simulink model "FuelCell5"  (R2016b)
settings: Solver=ode45  StartTime=0.0  StopTime=100.0  RelTol=1e-3
undefined symbols (not defined in the file): A, B, C, J, Jmax, lam, n, Rc, Tr
libraries: simulink x1
settings Model: Creator=Kelly  LastModifiedBy=Kelly

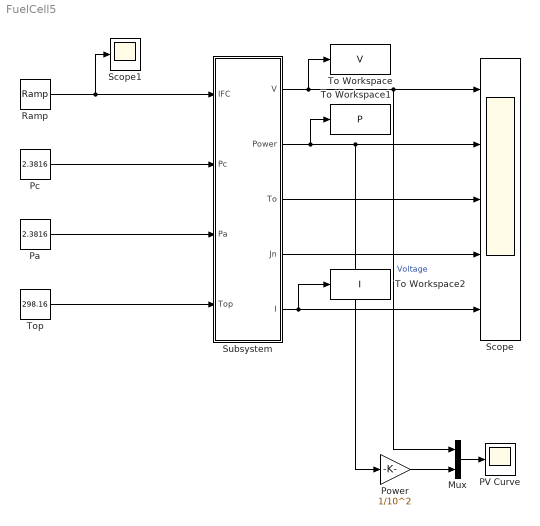
== system FuelCell5 ==
  Mux : Mux  Inputs=2
  PV Curve : Scope
  Pa : Constant  Value=2.3816
  Pc : Constant  Value=2.3816
  Power : Gain  Gain=1/10^2
  Ramp : simulink/Sources/Ramp  slope=Jmax*A/100  start=0  X0=J*A/100
  Scope : Scope  NumInputPorts=5
  Scope1 : Scope
  Subsystem : Subsystem
  To Workspace : ToWorkspace  VariableName=V  SaveFormat=Timeseries  SampleTime=-1
  To Workspace1 : ToWorkspace  VariableName=P  SaveFormat=Timeseries  SampleTime=-1
  To Workspace2 : ToWorkspace  VariableName=I  SaveFormat=Timeseries  SampleTime=-1
  Top : Constant  Value=298.16
  wires:
  Ramp/1 -> Scope1/1, Subsystem/1(IFC)
  Pc/1 -> Subsystem/2(Pc)
  Pa/1 -> Subsystem/3(Pa)
  Top/1 -> Subsystem/4(Top)
  Subsystem/1(V) -> To Workspace/1, Mux/1, Scope/1  "Voltage"
  Mux/1 -> PV Curve/1
  Power/1 -> Mux/2
  Subsystem/2(Power) -> To Workspace1/1, Power/1, Scope/2
  Subsystem/3(To) -> Scope/3
  Subsystem/4(Jn) -> Scope/4
  Subsystem/5(I) -> To Workspace2/1, Scope/5

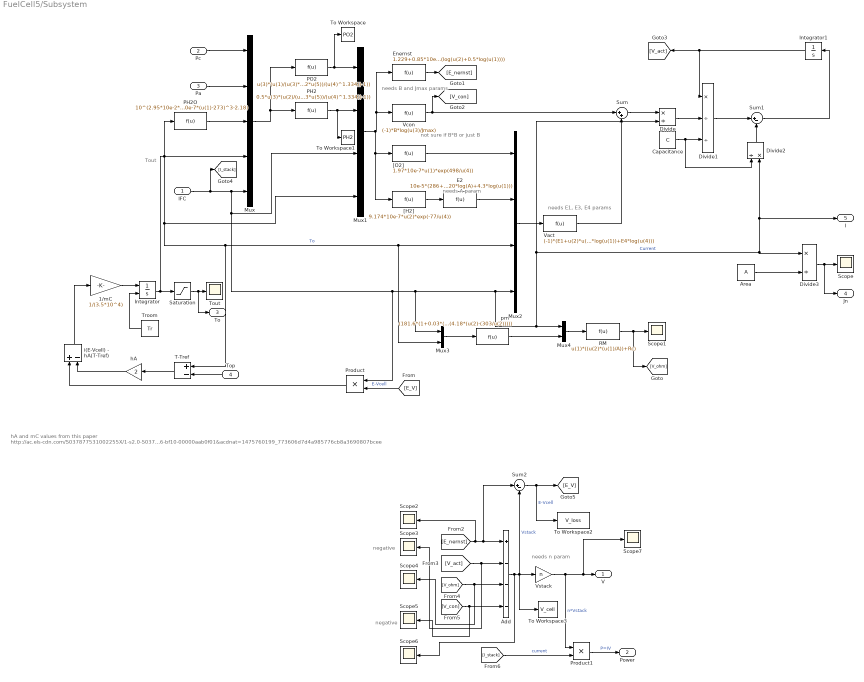
== system FuelCell5/Subsystem ==
  note: negative
  note: negative
  note: not sure if B*B or just B
  note: hA and mC values from this paper http://ac.els-cdn.com/S037877531002255X/1-s2.0-S037877531002255X-main.pdf?_tid=a0966334-8bc7-11e6-bf10-00000aab0f01&acdnat=1475760199_773606d7d4a985776cb8a3690807bcee
  note: Tout
  note: needs E1, E3, E4 params
  note: needs B and Jmax params
  note: needs A param
  note: needs n param
  IFC : Inport
  Pc : Inport  Port=2
  Pa : Inport  Port=3
  Top : Inport  Port=4
  1/mC : Gain  Gain=1/(3.5*10^4)
  Add : Sum  Inputs=+---
  Area : Constant  Value=A
  Capacitance : Constant  Value=C
  Divide : Product  Inputs=*/
  Divide1 : Product  Inputs=*//
  Divide2 : Product  Inputs=/*
  Divide3 : Product  Inputs=*/
  E2 : Fcn  Expr=10e-5*(286+20*log(A)+4.3*log(u(1)))
  Enernst : Fcn  Expr=1.229+0.85*10e-3*(u(4)-298.15)+4.3085*10e-5*(log(u(2)+0.5*log(u(1))))
  Integrator : Integrator  InitialConditionSource=external
  Integrator1 : Integrator
  Mux : Mux  Inputs=5
  Mux1 : Mux
  Mux2 : Mux
  Mux3 : Mux  Inputs=2
  Mux4 : Mux  Inputs=2
  PH2 : Fcn  Expr=0.5*u(3)*(u(2)/(u(3)*exp((1.653*u(5))/(u(4)^1.334))-1))
  PH2O : Fcn  Expr=10^(2.95*10e-2*(u(1)-273.15)-9.18*10e-5*(u(1)-273.15)^2+1.44*10e-7*(u(1)-273)^3-2.18)
  PO2 : Fcn  Expr=u(3)*(u(1)/(u(3)*exp((4.192*u(5))/(u(4)^1.334))-1))
  Product : Product
  Product1 : Product
  RM : Fcn  Expr=u(1)*((u(2)*(u(1)/A))+Rc)
  Saturation : Saturate
  Scope{,1..7} (8 alike) : Scope
  Sum : Sum  Inputs=|++
  Sum1 : Sum  Inputs=|+-
  Sum2 : Sum  Inputs=|+-
  T-Tref : Sum  Inputs=+-
  To Workspace : ToWorkspace  VariableName=PO2  SaveFormat=Timeseries  SampleTime=-1
  To Workspace1 : ToWorkspace  VariableName=PH2  SaveFormat=Timeseries  SampleTime=-1
  To Workspace2 : ToWorkspace  VariableName=V_loss  SaveFormat=Timeseries  SampleTime=-1
  To Workspace3 : ToWorkspace  VariableName=V_cell  SaveFormat=Timeseries  SampleTime=-1
  Tout : Scope
  Troom : Constant  Value=Tr
  Vact : Fcn  Expr=(-1)*(E1+u(2)*u(3)+E3*u(3)*log(u(1))+E4*log(u(4)))
  Vcon : Fcn  Expr=(-1)*B*log(u(3)/Jmax)
  Vstack : Gain  Gain=n
  "[H2]" : Fcn  Expr=9.174*10e-7*u(2)*exp(-77/u(4))
  "[O2]" : Fcn  Expr=1.97*10e-7*u(1)*exp(498/u(4))
  hA : Gain  Gain=2
  i(E-Vcell) - hA(T-Tref) : Sum  Inputs=+-
  pm : Fcn  Expr=(181.6*(1+0.03*(u(1)/A)+0.062*(u(2)/303)*(u(1)/A)^2.5))/((lam-0.634-3*(u(1)/A))*exp(4.18*(u(2)-(303/u(2)))))
  V : Outport
  Power : Outport  Port=2
  To : Outport  Port=3
  Jn : Outport  Port=4
  I : Outport  Port=5
  wires:
  Sum/1 -> Divide/1
  Divide/1 -> Divide1/2
  Sum1/1 -> Integrator1/1
  Integrator1/1 -> Divide1/1, [V_act]
  Capacitance/1 -> Divide2/1, Divide1/3
  [V_act] -> Scope3/1, Add/2
  [E_nernst] -> Scope2/1, Sum2/1, Add/1
  Product1/1 -> Power/1  "P=IV"
  [E_V] -> Product/2  "E-Vcell"
  [V_ohm] -> Scope4/1, Add/3
  Mux1/1 -> "[H2]"/1, "[O2]"/1, Enernst/1, Vcon/1
  Add/1 -> Scope6/1, To Workspace3/1, Sum2/2, Vstack/1  "Vstack"
  "[H2]"/1 -> E2/1
  Mux2/1 -> Vact/1
  [I_stack] -> Product1/2  "current"
  Sum2/1 -> To Workspace2/1, [E_V]  "E-Vcell"
  Top/1 -> T-Tref/2
  T-Tref/1 -> hA/1
  Mux/1 -> PH2/1, PO2/1
  "[O2]"/1 -> Mux2/1
  Pa/1 -> Mux/2
  PH2/1 -> To Workspace1/1, Mux1/2
  Vstack/1 -> Scope7/1, V/1, Product1/1  "n*Vstack"
  E2/1 -> Mux2/2
  IFC/1 -> [I_stack], Product/1, Mux3/1, I/1, Divide2/2, Divide3/1, Divide/2, Mux4/1, Mux2/4, Mux1/3, Mux/5  "Current"
  PH2O/1 -> Mux/3
  Pc/1 -> Mux/1
  Integrator/1 -> T-Tref/1, Mux3/2, Mux2/3, Mux1/4, PH2O/1, Mux/4, Saturation/1  "To"
  PO2/1 -> To Workspace/1, Mux1/1
  Vcon/1 -> [V_con], Sum/1
  [V_con] -> Scope5/1, Add/4
  Saturation/1 -> To/1, Tout/1
  1/mC/1 -> Integrator/1
  pm/1 -> Mux4/2
  Mux4/1 -> RM/1
  Troom/1 -> Integrator/2
  hA/1 -> i(E-Vcell) - hA(T-Tref)/2
  Product/1 -> i(E-Vcell) - hA(T-Tref)/1
  i(E-Vcell) - hA(T-Tref)/1 -> 1/mC/1
  Mux3/1 -> pm/1
  RM/1 -> [V_ohm], Scope1/1
  Divide2/1 -> Sum1/2
  Area/1 -> Divide3/2
  Enernst/1 -> [E_nernst]
  Divide3/1 -> Jn/1, Scope/1
  Divide1/1 -> Sum1/1
  Vact/1 -> Sum/2
